simulink model "SetResetWait_tmp"  (Simulink 8.3)
settings: Solver=ode45  StartTime=0.0  StopTime=10.0  RelTol=1e-3
settings Model: Creator=scaife  LastModifiedBy=bourbouh  CovSFcnEnable=on  ExtModeAutoUpdateStatusClock=off
settings DataIOCC: SignalLoggingName=sigsOut
settings DebuggingCC: SaveWithParameterizedLinksMsg=none  SignalResolutionControl=TryResolveAllWithWarning  SolverPrmCheckMsg=none  MultiTaskDSMMsg=warning  MultiTaskCondExecSysMsg=none  FrameProcessingCompatibilityMsg=error  StateNameClashWarn=none  StrictBusMsg=None
settings HardwareCC: TargetUnknown=on
settings SFSimCC: SimParseCustomCode=off
settings GRTTargetCC: GeneratePreprocessorConditionals=Use local settings

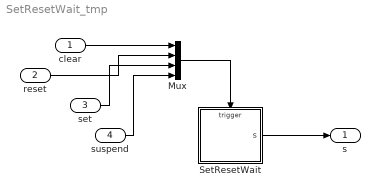
== system SetResetWait_tmp ==
  clear : Inport
  reset : Inport  Port=2
  set : Inport  Port=3
  suspend : Inport  Port=4
  Mux : Mux
  SetResetWait : Stateflow chart  TreatAsAtomicUnit=on
      settings: PermitHierarchicalResolution=ParametersOnly
  s : Outport
  wires:
  clear/1 -> Mux/1
  reset/1 -> Mux/2
  set/1 -> Mux/3
  suspend/1 -> Mux/4
  Mux/1 -> SetResetWait/Trigger
  SetResetWait/1(s) -> s/1

== stateflow chart SetResetWait ==
  state On
    en : s = 1
  state Off
    en : s = 3
  state Wait
    en : s = 2
  On -> Wait [order 1] : Suspend
  Off -> On [order 1] : Set
  On -> Off [order 2] : Reset
  Off -> Wait [order 2] : Suspend
  Wait -> Off : Clear
  (default) -> Off
  data: s output double
  events: Clear input EITHER_EDGE_EVENT; Reset input EITHER_EDGE_EVENT; Suspend input EITHER_EDGE_EVENT; Set input EITHER_EDGE_EVENT
